simulink model "DYNctl_ver4_etud_nonlineaire_plaque"  (R2014b)
settings: Solver=ode45  StartTime=0.0  StopTime=tfin  FixedStep=0.001  RelTol=1e-09
values from neighbouring files (symbols this model uses):
  ae = sym('ae',[4 1])    [MatlabProjet.m]    (also in bancEssaiConstantes.m = [1.3463 349.0774 1450.3848 703344.2113]; bancessai_ini.m)
  as = sym('as',[4 1])    [MatlabProjet.m]    (also in bancEssaiConstantes.m = [0.052961 30.5716 -1152.4168 344545.4587]; bancessai_ini.m)
  b_E1 = 13.029359254409743    (= 13.0293592544)    [MatlabProjet.m]    (also in bancEssaiConstantes.m; bancessai_ini.m)
  g = 9.81    [MatlabProjet.m]    (also in bancEssaiConstantes.m; bancessai_ini.m; trajectoire.m = sqrt(1 + dy.^2))
  Ixy = 0.0011691    [MatlabProjet.m]    (also in bancEssaiConstantes.m; bancessai_ini.m)
  L_bobine = 115    [MatlabProjet.m]    (also in bancEssaiConstantes.m = 0.115; bancessai_ini.m)
  mS = 0.0080*sig    [bancEssaiConstantes.m]
  mtot = mP + sig*mS    [bancEssaiConstantes.m]
  Pzeq = .015    (= 0.015)    [run_bancessai.m]
  R_bobine = 3.6    [MatlabProjet.m]    (also in bancEssaiConstantes.m; bancessai_ini.m)
  rABC = 95.20e-03    (= 0.0952)    [bancEssaiConstantes.m]
  Va_eq = R_bobine * Ia_eq    [MatlabEquilibre.m]    (also in bancessai_ini.m = Ia_eq*R_bobine; equilibre.m = Ia_eq*R_bobine)
  Vb_eq = R_bobine * Ib_eq    [MatlabEquilibre.m]    (also in bancessai_ini.m = Ib_eq*R_bobine; equilibre.m = Ib_eq*R_bobine)
  Vc_eq = R_bobine * Ic_eq    [MatlabEquilibre.m]    (also in bancessai_ini.m = Ic_eq*R_bobine; equilibre.m = Ic_eq*R_bobine)
  XA = r_ABC    (= 0.0952)    [MatlabProjet.m]    (also in bancEssaiConstantes.m; bancessai_ini.m)
  XB = -r_ABC*sind(30)    [MatlabProjet.m]    (also in bancEssaiConstantes.m = -rABC*sind(30); bancessai_ini.m)
  XC = XB    [MatlabProjet.m]    (also in bancEssaiConstantes.m = -rABC*sind(30); bancessai_ini.m)
  XD = r_DEF*sind(30)    [MatlabProjet.m]    (also in bancEssaiConstantes.m = +rDEF*sind(30); bancessai_ini.m)
  XE = -r_DEF    (= -0.08)    [MatlabProjet.m]    (also in bancEssaiConstantes.m; bancessai_ini.m)
  XF = XD    [MatlabProjet.m]    (also in bancEssaiConstantes.m = +rDEF*sind(30); bancessai_ini.m)
  YA = 0    [MatlabProjet.m]    (also in bancEssaiConstantes.m; bancessai_ini.m)
  YB = r_ABC*cosd(30)    [MatlabProjet.m]    (also in bancEssaiConstantes.m = +rABC*cosd(30); bancessai_ini.m)
  YC = -YB    [MatlabProjet.m]    (also in bancEssaiConstantes.m = -rABC*cosd(30); bancessai_ini.m)
  YD = r_DEF*cosd(30)    [MatlabProjet.m]    (also in bancEssaiConstantes.m = +rDEF*cosd(30); bancessai_ini.m)
  YE = 0    [MatlabProjet.m]    (also in bancEssaiConstantes.m; bancessai_ini.m)
  YF = -YD    [MatlabProjet.m]    (also in bancEssaiConstantes.m = -rDEF*cosd(30); bancessai_ini.m)
undefined symbols (not defined in the file or in its folder): den_pt, den_z, num_pt, num_z, sym2poly
settings Model: Creator=delafontaine  LastModifiedBy=lemg2013
settings SolverCC: AlgebraicLoopSolver=LineSearch
settings DataIOCC: SignalLoggingSaveFormat=ModelDataLogs
settings DebuggingCC: UnderspecifiedInitializationDetection=Classic  MergeDetectMultiDrivingBlocksExec=none  SolverPrmCheckMsg=none  MultiTaskDSMMsg=warning  MultiTaskCondExecSysMsg=none  FrameProcessingCompatibilityMsg=error
settings RTWCC: IncludeERTFirstTime=on

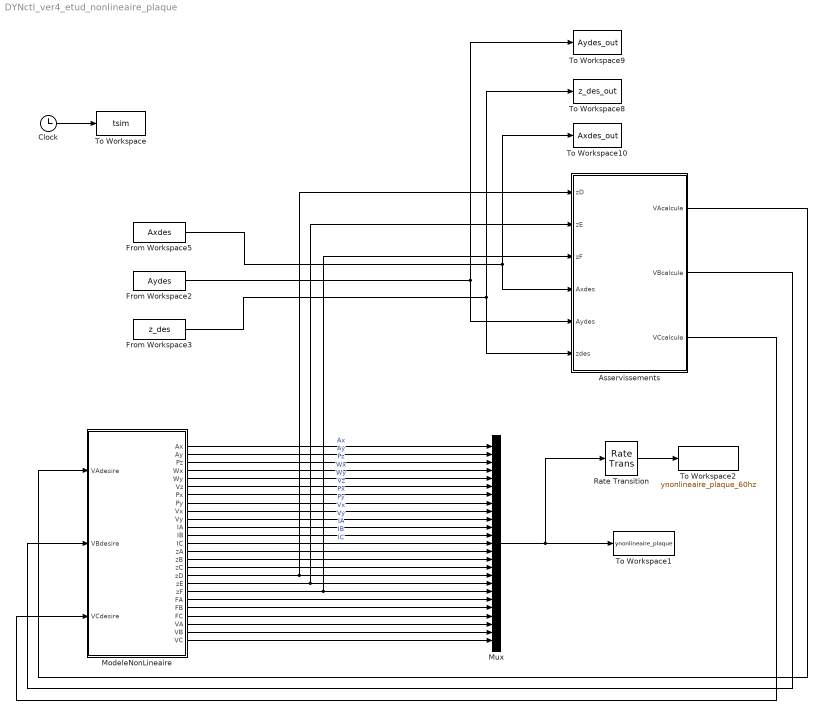
== system DYNctl_ver4_etud_nonlineaire_plaque ==
  Asservissements : Subsystem
      mask help: Simulink:masks:GenSFuncDesc_MD
      mask Help: eval('feval(''rtwprivate'',''rtwhelpview'',''rtw_sfcn_block'')');
  Clock : Clock
  From Workspace2 : FromWorkspace  VariableName=Aydes  SampleTime=0  Interpolate=off  OutputAfterFinalValue=Holding final value
  From Workspace3 : FromWorkspace  VariableName=z_des  SampleTime=0  Interpolate=off  OutputAfterFinalValue=Holding final value
  From Workspace5 : FromWorkspace  VariableName=Axdes  SampleTime=0  Interpolate=off  OutputAfterFinalValue=Holding final value
  ModeleNonLineaire : Subsystem
      mask help: Simulink:masks:GenSFuncDesc_MD
      mask Help: eval('feval(''rtwprivate'',''rtwhelpview'',''rtw_sfcn_block'')');
  Mux : Mux  Inputs=25
  Rate Transition : RateTransition  OutPortSampleTime=1/60
  To Workspace : ToWorkspace  VariableName=tsim  SampleTime=-1
  To Workspace1 : ToWorkspace  VariableName=ynonlineaire_plaque  SampleTime=-1
  To Workspace10 : ToWorkspace  VariableName=Axdes_out  SampleTime=-1
  To Workspace2 : ToWorkspace  VariableName=ynonlineaire_plaque_60hz  SampleTime=-1
  To Workspace8 : ToWorkspace  VariableName=z_des_out  SampleTime=-1
  To Workspace9 : ToWorkspace  VariableName=Aydes_out  SampleTime=-1
  wires:
  Clock/1 -> To Workspace/1
  From Workspace5/1 -> Asservissements/4(Axdes), To Workspace10/1
  ModeleNonLineaire/1(Ax) -> Mux/1  "Ax"
  ModeleNonLineaire/2(Ay) -> Mux/2  "Ay"
  ModeleNonLineaire/3(Pz) -> Mux/3  "Pz"
  ModeleNonLineaire/4(Wx) -> Mux/4  "Wx"
  ModeleNonLineaire/5(Wy) -> Mux/5  "Wy"
  ModeleNonLineaire/6(Vz) -> Mux/6  "Vz"
  ModeleNonLineaire/7(Px) -> Mux/7  "Px"
  ModeleNonLineaire/8(Py) -> Mux/8  "Py"
  ModeleNonLineaire/9(Vx) -> Mux/9  "Vx"
  ModeleNonLineaire/10(Vy) -> Mux/10  "Vy"
  ModeleNonLineaire/11(IA) -> Mux/11  "IA"
  ModeleNonLineaire/12(IB) -> Mux/12  "IB"
  ModeleNonLineaire/13(IC) -> Mux/13  "IC"
  From Workspace3/1 -> Asservissements/6(zdes), To Workspace8/1
  From Workspace2/1 -> Asservissements/5(Aydes), To Workspace9/1
  ModeleNonLineaire/20(FA) -> Mux/20
  ModeleNonLineaire/21(FB) -> Mux/21
  ModeleNonLineaire/22(FC) -> Mux/22
  ModeleNonLineaire/23(VA) -> Mux/23
  ModeleNonLineaire/24(VB) -> Mux/24
  ModeleNonLineaire/25(VC) -> Mux/25
  ModeleNonLineaire/17(zD) -> Asservissements/1(zD), Mux/17
  ModeleNonLineaire/18(zE) -> Asservissements/2(zE), Mux/18
  ModeleNonLineaire/19(zF) -> Asservissements/3(zF), Mux/19
  ModeleNonLineaire/14(zA) -> Mux/14
  ModeleNonLineaire/15(zB) -> Mux/15
  ModeleNonLineaire/16(zC) -> Mux/16
  Asservissements/1(VAcalcule) -> ModeleNonLineaire/1(VAdesire)
  Asservissements/2(VBcalcule) -> ModeleNonLineaire/2(VBdesire)
  Asservissements/3(VCcalcule) -> ModeleNonLineaire/3(VCdesire)
  Mux/1 -> Rate Transition/1, To Workspace1/1
  Rate Transition/1 -> To Workspace2/1

== system DYNctl_ver4_etud_nonlineaire_plaque/Asservissements ==
  zD : Inport
  zE : Inport  Port=2
  zF : Inport  Port=3
  Axdes : Inport  Port=4
  Aydes : Inport  Port=5
  zdes : Inport  Port=6
  Asservissements_fc : Subsystem
  __InputSSForSFun__ : Subsystem
  __OutputSSForSFun__ : Subsystem
  VAcalcule : Outport
  VBcalcule : Outport  Port=2
  VCcalcule : Outport  Port=3
  wires:
  zD/1 -> __InputSSForSFun__/1(zD)
  zE/1 -> __InputSSForSFun__/2(zE)
  zF/1 -> __InputSSForSFun__/3(zF)
  Axdes/1 -> __InputSSForSFun__/4(Axdes)
  Aydes/1 -> __InputSSForSFun__/5(Aydes)
  zdes/1 -> __InputSSForSFun__/6(zdes)
  __InputSSForSFun__/1(__UniqueOutportName__1__) -> Asservissements_fc/1(zD)
  __InputSSForSFun__/2(__UniqueOutportName__2__) -> Asservissements_fc/2(zE)
  __InputSSForSFun__/3(__UniqueOutportName__3__) -> Asservissements_fc/3(zF)
  __InputSSForSFun__/4(__UniqueOutportName__4__) -> Asservissements_fc/4(Axdes)
  __InputSSForSFun__/5(__UniqueOutportName__5__) -> Asservissements_fc/5(Aydes)
  __InputSSForSFun__/6(__UniqueOutportName__6__) -> Asservissements_fc/6(zdes)
  Asservissements_fc/1(Vacalc) -> __OutputSSForSFun__/1(__UniqueInportName__1__)
  Asservissements_fc/2(Vbcalc) -> __OutputSSForSFun__/2(__UniqueInportName__2__)
  Asservissements_fc/3(Vccalc) -> __OutputSSForSFun__/3(__UniqueInportName__3__)
  __OutputSSForSFun__/1(VAcalcule) -> VAcalcule/1
  __OutputSSForSFun__/2(VBcalcule) -> VBcalcule/1
  __OutputSSForSFun__/3(VCcalcule) -> VCcalcule/1

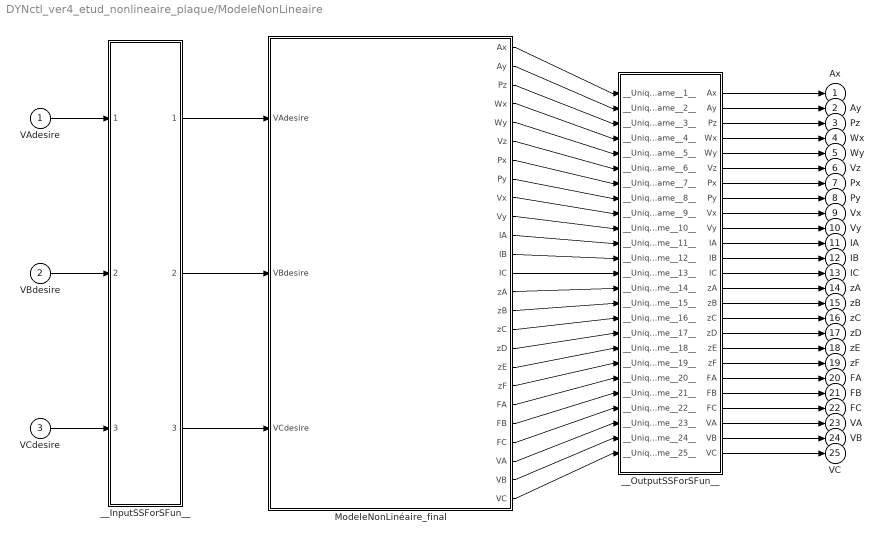
== system DYNctl_ver4_etud_nonlineaire_plaque/ModeleNonLineaire ==
  VAdesire : Inport
  VBdesire : Inport  Port=2
  VCdesire : Inport  Port=3
  ModeleNonLinéaire_final : Subsystem
  __InputSSForSFun__ : Subsystem
  __OutputSSForSFun__ : Subsystem
  Ax : Outport
  Ay : Outport  Port=2
  Pz : Outport  Port=3
  Wx : Outport  Port=4
  Wy : Outport  Port=5
  Vz : Outport  Port=6
  Px : Outport  Port=7
  Py : Outport  Port=8
  Vx : Outport  Port=9
  Vy : Outport  Port=10
  IA : Outport  Port=11
  IB : Outport  Port=12
  IC : Outport  Port=13
  zA : Outport  Port=14
  zB : Outport  Port=15
  zC : Outport  Port=16
  zD : Outport  Port=17
  zE : Outport  Port=18
  zF : Outport  Port=19
  FA : Outport  Port=20
  FB : Outport  Port=21
  FC : Outport  Port=22
  VA : Outport  Port=23
  VB : Outport  Port=24
  VC : Outport  Port=25
  wires:
  VAdesire/1 -> __InputSSForSFun__/1(VAdesire)
  VBdesire/1 -> __InputSSForSFun__/2(VBdesire)
  VCdesire/1 -> __InputSSForSFun__/3(VCdesire)
  __InputSSForSFun__/1(__UniqueOutportName__1__) -> ModeleNonLinéaire_final/1(VAdesire)
  ModeleNonLinéaire_final/1(Ax) -> __OutputSSForSFun__/1(__UniqueInportName__1__)
  ModeleNonLinéaire_final/2(Ay) -> __OutputSSForSFun__/2(__UniqueInportName__2__)
  ModeleNonLinéaire_final/3(Pz) -> __OutputSSForSFun__/3(__UniqueInportName__3__)
  ModeleNonLinéaire_final/4(Wx) -> __OutputSSForSFun__/4(__UniqueInportName__4__)
  ModeleNonLinéaire_final/5(Wy) -> __OutputSSForSFun__/5(__UniqueInportName__5__)
  ModeleNonLinéaire_final/6(Vz) -> __OutputSSForSFun__/6(__UniqueInportName__6__)
  ModeleNonLinéaire_final/7(Px) -> __OutputSSForSFun__/7(__UniqueInportName__7__)
  ModeleNonLinéaire_final/8(Py) -> __OutputSSForSFun__/8(__UniqueInportName__8__)
  ModeleNonLinéaire_final/9(Vx) -> __OutputSSForSFun__/9(__UniqueInportName__9__)
  ModeleNonLinéaire_final/10(Vy) -> __OutputSSForSFun__/10(__UniqueInportName__10__)
  ModeleNonLinéaire_final/11(IA) -> __OutputSSForSFun__/11(__UniqueInportName__11__)
  ModeleNonLinéaire_final/12(IB) -> __OutputSSForSFun__/12(__UniqueInportName__12__)
  ModeleNonLinéaire_final/13(IC) -> __OutputSSForSFun__/13(__UniqueInportName__13__)
  ModeleNonLinéaire_final/14(zA) -> __OutputSSForSFun__/14(__UniqueInportName__14__)
  ModeleNonLinéaire_final/15(zB) -> __OutputSSForSFun__/15(__UniqueInportName__15__)
  ModeleNonLinéaire_final/16(zC) -> __OutputSSForSFun__/16(__UniqueInportName__16__)
  ModeleNonLinéaire_final/17(zD) -> __OutputSSForSFun__/17(__UniqueInportName__17__)
  ModeleNonLinéaire_final/18(zE) -> __OutputSSForSFun__/18(__UniqueInportName__18__)
  ModeleNonLinéaire_final/19(zF) -> __OutputSSForSFun__/19(__UniqueInportName__19__)
  ModeleNonLinéaire_final/20(FA) -> __OutputSSForSFun__/20(__UniqueInportName__20__)
  ModeleNonLinéaire_final/21(FB) -> __OutputSSForSFun__/21(__UniqueInportName__21__)
  ModeleNonLinéaire_final/22(FC) -> __OutputSSForSFun__/22(__UniqueInportName__22__)
  ModeleNonLinéaire_final/23(VA) -> __OutputSSForSFun__/23(__UniqueInportName__23__)
  ModeleNonLinéaire_final/24(VB) -> __OutputSSForSFun__/24(__UniqueInportName__24__)
  ModeleNonLinéaire_final/25(VC) -> __OutputSSForSFun__/25(__UniqueInportName__25__)
  __OutputSSForSFun__/1(Ax) -> Ax/1
  __OutputSSForSFun__/2(Ay) -> Ay/1
  __OutputSSForSFun__/3(Pz) -> Pz/1
  __OutputSSForSFun__/4(Wx) -> Wx/1
  __OutputSSForSFun__/5(Wy) -> Wy/1
  __OutputSSForSFun__/6(Vz) -> Vz/1
  __OutputSSForSFun__/7(Px) -> Px/1
  __OutputSSForSFun__/8(Py) -> Py/1
  __OutputSSForSFun__/9(Vx) -> Vx/1
  __OutputSSForSFun__/10(Vy) -> Vy/1
  __OutputSSForSFun__/11(IA) -> IA/1
  __OutputSSForSFun__/12(IB) -> IB/1
  __OutputSSForSFun__/13(IC) -> IC/1
  __OutputSSForSFun__/14(zA) -> zA/1
  __OutputSSForSFun__/15(zB) -> zB/1
  __OutputSSForSFun__/16(zC) -> zC/1
  __OutputSSForSFun__/17(zD) -> zD/1
  __OutputSSForSFun__/18(zE) -> zE/1
  __OutputSSForSFun__/19(zF) -> zF/1
  __OutputSSForSFun__/20(FA) -> FA/1
  __OutputSSForSFun__/21(FB) -> FB/1
  __OutputSSForSFun__/22(FC) -> FC/1
  __OutputSSForSFun__/23(VA) -> VA/1
  __OutputSSForSFun__/24(VB) -> VB/1
  __OutputSSForSFun__/25(VC) -> VC/1
  __InputSSForSFun__/2(__UniqueOutportName__2__) -> ModeleNonLinéaire_final/2(VBdesire)
  __InputSSForSFun__/3(__UniqueOutportName__3__) -> ModeleNonLinéaire_final/3(VCdesire)

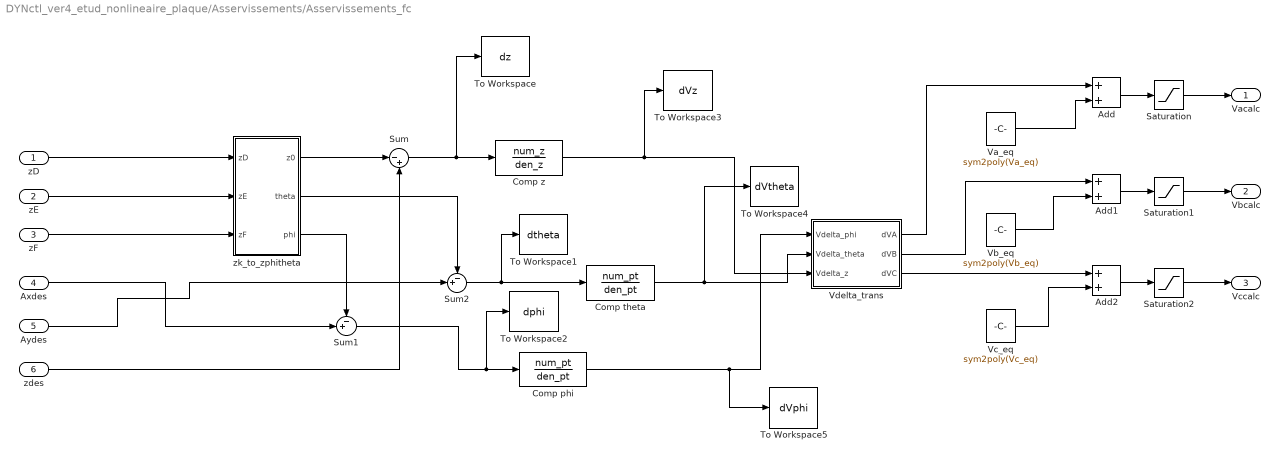
== system DYNctl_ver4_etud_nonlineaire_plaque/Asservissements/Asservissements_fc ==
  zD : Inport
  zE : Inport  Port=2
  zF : Inport  Port=3
  Axdes : Inport  Port=4
  Aydes : Inport  Port=5
  zdes : Inport  Port=6
  Add : Sum
  Add1 : Sum
  Add2 : Sum
  Comp phi : TransferFcn  Numerator=num_pt  Denominator=den_pt
  Comp theta : TransferFcn  Numerator=num_pt  Denominator=den_pt
  Comp z : TransferFcn  Numerator=num_z  Denominator=den_z
  Saturation : Saturate  UpperLimit=22  LowerLimit=-22
  Saturation1 : Saturate  UpperLimit=22  LowerLimit=-22
  Saturation2 : Saturate  UpperLimit=22  LowerLimit=-22
  Sum : Sum  Inputs=|-+
  Sum1 : Sum  Inputs=-+|
  Sum2 : Sum  Inputs=-+|
  To Workspace : ToWorkspace  VariableName=dz  SampleTime=-1
      settings: Save2DSignal=2-D array (concatenate along first dimension)
  To Workspace1 : ToWorkspace  VariableName=dtheta  SampleTime=-1
      settings: Save2DSignal=2-D array (concatenate along first dimension)
  To Workspace2 : ToWorkspace  VariableName=dphi  SampleTime=-1
      settings: Save2DSignal=2-D array (concatenate along first dimension)
  To Workspace3 : ToWorkspace  VariableName=dVz  SampleTime=-1
      settings: Save2DSignal=2-D array (concatenate along first dimension)
  To Workspace4 : ToWorkspace  VariableName=dVtheta  SampleTime=-1
      settings: Save2DSignal=2-D array (concatenate along first dimension)
  To Workspace5 : ToWorkspace  VariableName=dVphi  SampleTime=-1
      settings: Save2DSignal=2-D array (concatenate along first dimension)
  Va_eq : Constant  Value=sym2poly(Va_eq)  VectorParams1D=off
  Vb_eq : Constant  Value=sym2poly(Vb_eq)  VectorParams1D=off
  Vc_eq : Constant  Value=sym2poly(Vc_eq)  VectorParams1D=off
  Vdelta_trans : Subsystem
  zk_to_zphitheta : Subsystem
  Vacalc : Outport
  Vbcalc : Outport  Port=2
  Vccalc : Outport  Port=3
  wires:
  zD/1 -> zk_to_zphitheta/1(zD)
  zE/1 -> zk_to_zphitheta/2(zE)
  zF/1 -> zk_to_zphitheta/3(zF)
  zdes/1 -> Sum/2
  zk_to_zphitheta/1(z0) -> Sum/1
  Sum/1 -> To Workspace/1, Comp z/1
  Comp z/1 -> To Workspace3/1, Vdelta_trans/3(Vdelta_z)
  zk_to_zphitheta/3(phi) -> Sum1/1
  zk_to_zphitheta/2(theta) -> Sum2/1
  Vdelta_trans/3(dVC) -> Add2/1
  Sum1/1 -> Comp phi/1, To Workspace2/1
  Sum2/1 -> To Workspace1/1, Comp theta/1
  Comp phi/1 -> To Workspace5/1, Vdelta_trans/1(Vdelta_phi)
  Vdelta_trans/1(dVA) -> Add/1
  Vdelta_trans/2(dVB) -> Add1/1
  Comp theta/1 -> To Workspace4/1, Vdelta_trans/2(Vdelta_theta)
  Add/1 -> Saturation/1
  Add1/1 -> Saturation1/1
  Add2/1 -> Saturation2/1
  Va_eq/1 -> Add/2
  Vc_eq/1 -> Add2/2
  Vb_eq/1 -> Add1/2
  Axdes/1 -> Sum1/2
  Aydes/1 -> Sum2/2
  Saturation/1 -> Vacalc/1
  Saturation1/1 -> Vbcalc/1
  Saturation2/1 -> Vccalc/1

== system DYNctl_ver4_etud_nonlineaire_plaque/Asservissements/__InputSSForSFun__ ==
  zD : Inport
  zE : Inport  Port=2
  zF : Inport  Port=3
  Axdes : Inport  Port=4
  Aydes : Inport  Port=5
  zdes : Inport  Port=6
  __UniqueOutportName__1__ : Outport
  __UniqueOutportName__2__ : Outport  Port=2
  __UniqueOutportName__3__ : Outport  Port=3
  __UniqueOutportName__4__ : Outport  Port=4
  __UniqueOutportName__5__ : Outport  Port=5
  __UniqueOutportName__6__ : Outport  Port=6
  wires:
  zD/1 -> __UniqueOutportName__1__/1
  zE/1 -> __UniqueOutportName__2__/1
  zF/1 -> __UniqueOutportName__3__/1
  Axdes/1 -> __UniqueOutportName__4__/1
  Aydes/1 -> __UniqueOutportName__5__/1
  zdes/1 -> __UniqueOutportName__6__/1

== system DYNctl_ver4_etud_nonlineaire_plaque/Asservissements/__OutputSSForSFun__ ==
  __UniqueInportName__1__ : Inport
  __UniqueInportName__2__ : Inport  Port=2
  __UniqueInportName__3__ : Inport  Port=3
  VAcalcule : Outport
  VBcalcule : Outport  Port=2
  VCcalcule : Outport  Port=3
  wires:
  __UniqueInportName__1__/1 -> VAcalcule/1
  __UniqueInportName__2__/1 -> VBcalcule/1
  __UniqueInportName__3__/1 -> VCcalcule/1

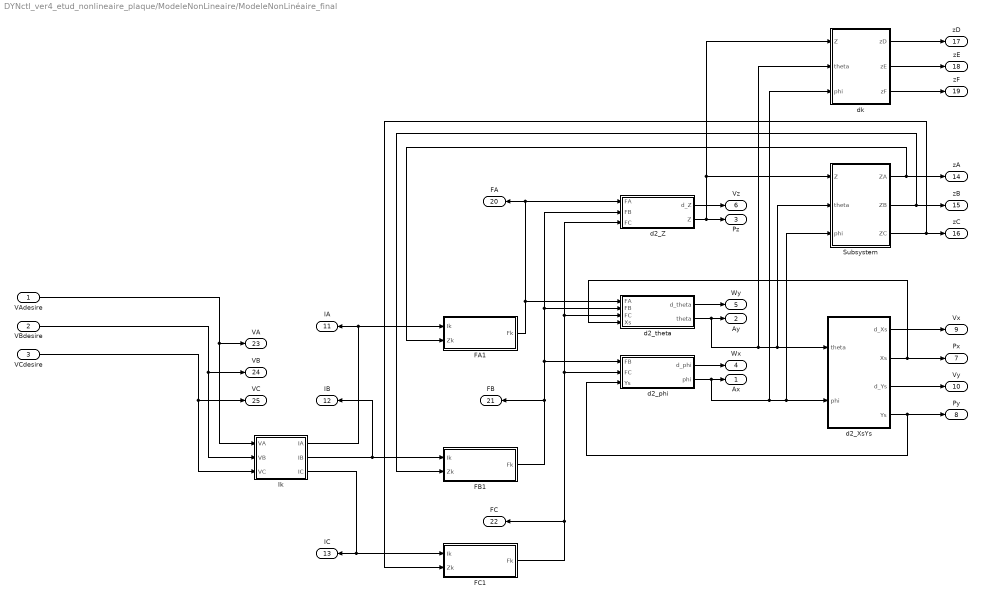
== system DYNctl_ver4_etud_nonlineaire_plaque/ModeleNonLineaire/ModeleNonLinéaire_final ==
  VAdesire : Inport
  VBdesire : Inport  Port=2
  VCdesire : Inport  Port=3
  FA1 : Subsystem
  FB1 : Subsystem
  FC1 : Subsystem
  Ik : Subsystem
  Subsystem : Subsystem
  d2_XsYs : Subsystem
  d2_Z : Subsystem
  d2_phi : Subsystem
  d2_theta : Subsystem
  dk : Subsystem
  Ax : Outport
  Ay : Outport  Port=2
  Pz : Outport  Port=3
  Wx : Outport  Port=4
  Wy : Outport  Port=5
  Vz : Outport  Port=6
  Px : Outport  Port=7
  Py : Outport  Port=8
  Vx : Outport  Port=9
  Vy : Outport  Port=10
  IA : Outport  Port=11
  IB : Outport  Port=12
  IC : Outport  Port=13
  zA : Outport  Port=14
  zB : Outport  Port=15
  zC : Outport  Port=16
  zD : Outport  Port=17
  zE : Outport  Port=18
  zF : Outport  Port=19
  FA : Outport  Port=20
  FB : Outport  Port=21
  FC : Outport  Port=22
  VA : Outport  Port=23
  VB : Outport  Port=24
  VC : Outport  Port=25
  wires:
  VAdesire/1 -> Ik/1(VA), VA/1
  VBdesire/1 -> VB/1, Ik/2(VB)
  VCdesire/1 -> Ik/3(VC), VC/1
  Ik/1(IA) -> IA/1, FA1/1(Ik)
  Ik/2(IB) -> IB/1, FB1/1(Ik)
  Ik/3(IC) -> FC1/1(Ik), IC/1
  FA1/1(Fk) -> FA/1, d2_Z/1(FA), d2_theta/1(FA)
  FB1/1(Fk) -> d2_phi/1(FB), d2_Z/2(FB), d2_theta/2(FB), FB/1
  FC1/1(Fk) -> d2_Z/3(FC), d2_theta/3(FC), d2_phi/2(FC), FC/1
  d2_phi/2("phi ") -> Ax/1, dk/3(phi), Subsystem/3(phi), d2_XsYs/2(phi)
  d2_theta/2("theta ") -> Ay/1, dk/2(theta), Subsystem/2(theta), d2_XsYs/1(theta)
  d2_XsYs/2(Xs) -> d2_theta/4(Xs), Px/1
  d2_XsYs/4(Ys) -> Py/1, d2_phi/3(Ys)
  d2_Z/2(Z) -> dk/1(Z), Subsystem/1(Z), Pz/1
  Subsystem/1(ZA) -> FA1/2(Zk), zA/1
  Subsystem/2(ZB) -> FB1/2(Zk), zB/1
  Subsystem/3(ZC) -> FC1/2(Zk), zC/1
  d2_phi/1("d_phi ") -> Wx/1
  d2_theta/1("d_theta ") -> Wy/1
  d2_Z/1(d_Z) -> Vz/1
  d2_XsYs/1(d_Xs) -> Vx/1
  d2_XsYs/3(d_Ys) -> Vy/1
  dk/1(zD) -> zD/1
  dk/2(zE) -> zE/1
  dk/3(zF) -> zF/1

== system DYNctl_ver4_etud_nonlineaire_plaque/ModeleNonLineaire/__InputSSForSFun__ ==
  VAdesire : Inport
  VBdesire : Inport  Port=2
  VCdesire : Inport  Port=3
  __UniqueOutportName__1__ : Outport
  __UniqueOutportName__2__ : Outport  Port=2
  __UniqueOutportName__3__ : Outport  Port=3
  wires:
  VAdesire/1 -> __UniqueOutportName__1__/1
  VBdesire/1 -> __UniqueOutportName__2__/1
  VCdesire/1 -> __UniqueOutportName__3__/1

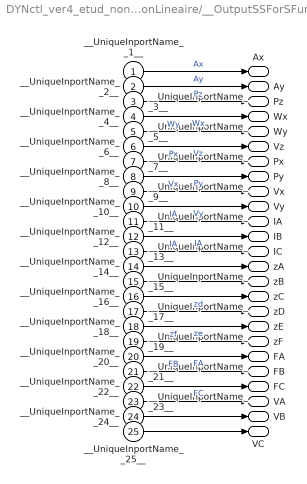
== system DYNctl_ver4_etud_nonlineaire_plaque/ModeleNonLineaire/__OutputSSForSFun__ ==
  __UniqueInportName__1__ : Inport
  __UniqueInportName__2__ : Inport  Port=2
  __UniqueInportName__3__ : Inport  Port=3
  __UniqueInportName__4__ : Inport  Port=4
  __UniqueInportName__5__ : Inport  Port=5
  __UniqueInportName__6__ : Inport  Port=6
  __UniqueInportName__7__ : Inport  Port=7
  __UniqueInportName__8__ : Inport  Port=8
  __UniqueInportName__9__ : Inport  Port=9
  __UniqueInportName__10__ : Inport  Port=10
  __UniqueInportName__11__ : Inport  Port=11
  __UniqueInportName__12__ : Inport  Port=12
  __UniqueInportName__13__ : Inport  Port=13
  __UniqueInportName__14__ : Inport  Port=14
  __UniqueInportName__15__ : Inport  Port=15
  __UniqueInportName__16__ : Inport  Port=16
  __UniqueInportName__17__ : Inport  Port=17
  __UniqueInportName__18__ : Inport  Port=18
  __UniqueInportName__19__ : Inport  Port=19
  __UniqueInportName__20__ : Inport  Port=20
  __UniqueInportName__21__ : Inport  Port=21
  __UniqueInportName__22__ : Inport  Port=22
  __UniqueInportName__23__ : Inport  Port=23
  __UniqueInportName__24__ : Inport  Port=24
  __UniqueInportName__25__ : Inport  Port=25
  Ax : Outport
  Ay : Outport  Port=2
  Pz : Outport  Port=3
  Wx : Outport  Port=4
  Wy : Outport  Port=5
  Vz : Outport  Port=6
  Px : Outport  Port=7
  Py : Outport  Port=8
  Vx : Outport  Port=9
  Vy : Outport  Port=10
  IA : Outport  Port=11
  IB : Outport  Port=12
  IC : Outport  Port=13
  zA : Outport  Port=14
  zB : Outport  Port=15
  zC : Outport  Port=16
  zD : Outport  Port=17
  zE : Outport  Port=18
  zF : Outport  Port=19
  FA : Outport  Port=20
  FB : Outport  Port=21
  FC : Outport  Port=22
  VA : Outport  Port=23
  VB : Outport  Port=24
  VC : Outport  Port=25
  wires:
  __UniqueInportName__1__/1 -> Ax/1  "Ax"
  __UniqueInportName__2__/1 -> Ay/1  "Ay"
  __UniqueInportName__3__/1 -> Pz/1  "Pz"
  __UniqueInportName__4__/1 -> Wx/1  "Wx"
  __UniqueInportName__5__/1 -> Wy/1  "Wy"
  __UniqueInportName__6__/1 -> Vz/1  "Vz"
  __UniqueInportName__7__/1 -> Px/1  "Px"
  __UniqueInportName__8__/1 -> Py/1  "Py"
  __UniqueInportName__9__/1 -> Vx/1  "Vx"
  __UniqueInportName__10__/1 -> Vy/1  "Vy"
  __UniqueInportName__11__/1 -> IA/1  "IA"
  __UniqueInportName__12__/1 -> IB/1  "IA"
  __UniqueInportName__13__/1 -> IC/1  "IA"
  __UniqueInportName__14__/1 -> zA/1
  __UniqueInportName__15__/1 -> zB/1
  __UniqueInportName__16__/1 -> zC/1
  __UniqueInportName__17__/1 -> zD/1  "zd"
  __UniqueInportName__18__/1 -> zE/1  "ze"
  __UniqueInportName__19__/1 -> zF/1  "zf"
  __UniqueInportName__20__/1 -> FA/1  "FA"
  __UniqueInportName__21__/1 -> FB/1  "FB"
  __UniqueInportName__22__/1 -> FC/1  "FC"
  __UniqueInportName__23__/1 -> VA/1
  __UniqueInportName__24__/1 -> VB/1
  __UniqueInportName__25__/1 -> VC/1

== system DYNctl_ver4_etud_nonlineaire_plaque/Asservissements/Asservissements_fc/Vdelta_trans ==
  Vdelta_phi : Inport
  Vdelta_theta : Inport  Port=2
  Vdelta_z : Inport  Port=3
  Demux : Demux  Outputs=3
  Mux : Mux  Inputs=3
  Product : Product  Multiplication=Matrix(*)
  u : Constant  Value=inv(u)  VectorParams1D=off
  dVA : Outport
  dVB : Outport  Port=2
  dVC : Outport  Port=3
  wires:
  u/1 -> Product/1
  Mux/1 -> Product/2
  Demux/1 -> dVA/1
  Demux/2 -> dVB/1
  Demux/3 -> dVC/1
  Product/1 -> Demux/1
  Vdelta_phi/1 -> Mux/1
  Vdelta_theta/1 -> Mux/2
  Vdelta_z/1 -> Mux/3

== system DYNctl_ver4_etud_nonlineaire_plaque/Asservissements/Asservissements_fc/zk_to_zphitheta ==
  zD : Inport
  zE : Inport  Port=2
  zF : Inport  Port=3
  Add : Sum  Inputs=+++
  Constant : Constant  Value=3
  Constant1 : Constant  Value=-XE
  Constant2 : Constant  Value=XD
  Constant3 : Constant  Value=YD
  Divide : Product  Inputs=*/
  Divide1 : Product  Inputs=*/
  Divide2 : Product  Inputs=*/
  Product : Product
  Sum : Sum  Inputs=|+-
  Sum1 : Sum  Inputs=|-++
  z0 : Outport
  theta : Outport  Port=2
  phi : Outport  Port=3
  wires:
  zD/1 -> Sum1/2, Add/1
  zE/1 -> Sum/1, Add/2
  zF/1 -> Add/3
  Add/1 -> Divide/1
  Constant/1 -> Divide/2
  Divide/1 -> Sum1/1, Sum/2, z0/1
  Sum/1 -> Divide1/1
  Constant1/1 -> Divide1/2
  Divide1/1 -> Product/1, theta/1
  Constant2/1 -> Product/2
  Product/1 -> Sum1/3
  Sum1/1 -> Divide2/1
  Constant3/1 -> Divide2/2
  Divide2/1 -> phi/1

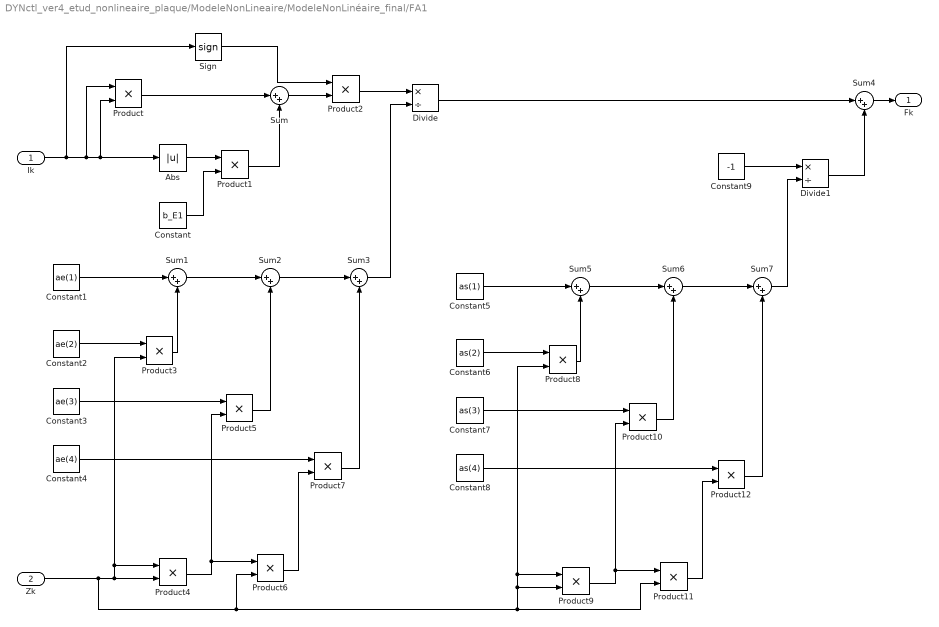
== system DYNctl_ver4_etud_nonlineaire_plaque/ModeleNonLineaire/ModeleNonLinéaire_final/FA1 ==
  Ik : Inport
  Zk : Inport  Port=2
  Abs : Abs
  Constant : Constant  Value=b_E1
  Constant1 : Constant  Value=ae(1)
  Constant2 : Constant  Value=ae(2)
  Constant3 : Constant  Value=ae(3)
  Constant4 : Constant  Value=ae(4)
  Constant5 : Constant  Value=as(1)
  Constant6 : Constant  Value=as(2)
  Constant7 : Constant  Value=as(3)
  Constant8 : Constant  Value=as(4)
  Constant9 : Constant  Value=-1
  Divide : Product  Inputs=*/
  Divide1 : Product  Inputs=*/
  Product{,1..12} (13 alike) : Product
  Sign : Signum
  Sum{,1..7} (8 alike) : Sum  Inputs=|++
  Fk : Outport
  wires:
  Ik/1 -> Sign/1, Product/1, Abs/1, Product/2
  Abs/1 -> Product1/1
  Constant/1 -> Product1/2
  Product1/1 -> Sum/2
  Product/1 -> Sum/1
  Sum/1 -> Product2/2
  Sign/1 -> Product2/1
  Constant1/1 -> Sum1/1
  Constant2/1 -> Product3/1
  Product3/1 -> Sum1/2
  Sum1/1 -> Sum2/1
  Product4/1 -> Product6/1, Product5/2
  Constant3/1 -> Product5/1
  Product5/1 -> Sum2/2
  Constant4/1 -> Product7/1
  Product6/1 -> Product7/2
  Product7/1 -> Sum3/2
  Sum2/1 -> Sum3/1
  Product2/1 -> Divide/1
  Sum3/1 -> Divide/2
  Constant5/1 -> Sum5/1
  Constant6/1 -> Product8/1
  Zk/1 -> Product11/2, Product8/2, Product9/1, Product9/2, Product6/2, Product3/2, Product4/1, Product4/2
  Product8/1 -> Sum5/2
  Sum5/1 -> Sum6/1
  Product9/1 -> Product11/1, Product10/2
  Constant7/1 -> Product10/1
  Product10/1 -> Sum6/2
  Constant8/1 -> Product12/1
  Product11/1 -> Product12/2
  Product12/1 -> Sum7/2
  Sum6/1 -> Sum7/1
  Sum7/1 -> Divide1/2
  Divide/1 -> Sum4/1
  Constant9/1 -> Divide1/1
  Divide1/1 -> Sum4/2
  Sum4/1 -> Fk/1

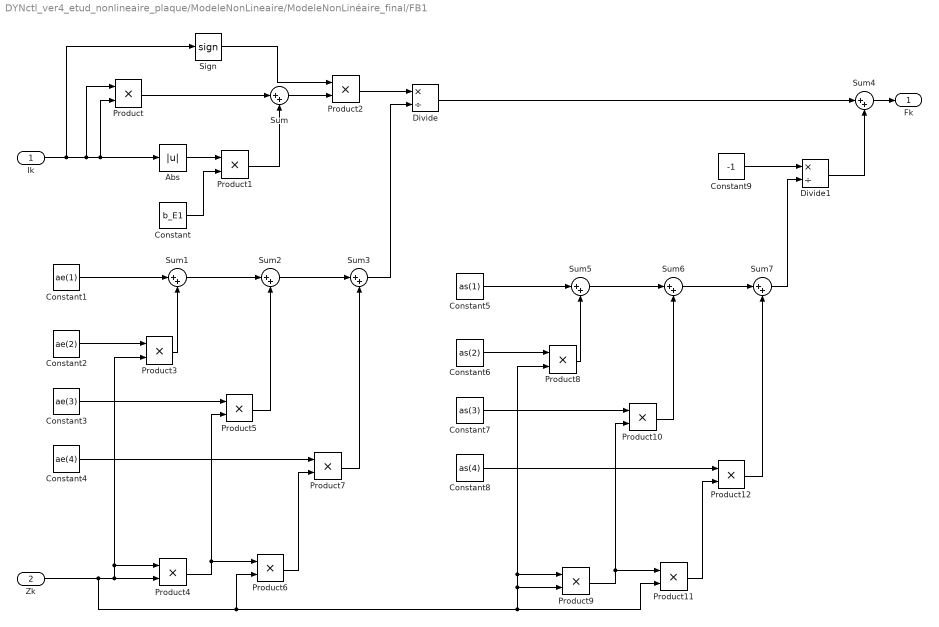
== system DYNctl_ver4_etud_nonlineaire_plaque/ModeleNonLineaire/ModeleNonLinéaire_final/FB1 ==
  Ik : Inport
  Zk : Inport  Port=2
  Abs : Abs
  Constant : Constant  Value=b_E1
  Constant1 : Constant  Value=ae(1)
  Constant2 : Constant  Value=ae(2)
  Constant3 : Constant  Value=ae(3)
  Constant4 : Constant  Value=ae(4)
  Constant5 : Constant  Value=as(1)
  Constant6 : Constant  Value=as(2)
  Constant7 : Constant  Value=as(3)
  Constant8 : Constant  Value=as(4)
  Constant9 : Constant  Value=-1
  Divide : Product  Inputs=*/
  Divide1 : Product  Inputs=*/
  Product{,1..12} (13 alike) : Product
  Sign : Signum
  Sum{,1..7} (8 alike) : Sum  Inputs=|++
  Fk : Outport
  wires:
  Ik/1 -> Sign/1, Product/1, Abs/1, Product/2
  Abs/1 -> Product1/1
  Constant/1 -> Product1/2
  Product1/1 -> Sum/2
  Product/1 -> Sum/1
  Sum/1 -> Product2/2
  Sign/1 -> Product2/1
  Constant1/1 -> Sum1/1
  Constant2/1 -> Product3/1
  Product3/1 -> Sum1/2
  Sum1/1 -> Sum2/1
  Product4/1 -> Product6/1, Product5/2
  Constant3/1 -> Product5/1
  Product5/1 -> Sum2/2
  Constant4/1 -> Product7/1
  Product6/1 -> Product7/2
  Product7/1 -> Sum3/2
  Sum2/1 -> Sum3/1
  Product2/1 -> Divide/1
  Sum3/1 -> Divide/2
  Constant5/1 -> Sum5/1
  Constant6/1 -> Product8/1
  Zk/1 -> Product11/2, Product8/2, Product9/1, Product9/2, Product6/2, Product3/2, Product4/1, Product4/2
  Product8/1 -> Sum5/2
  Sum5/1 -> Sum6/1
  Product9/1 -> Product11/1, Product10/2
  Constant7/1 -> Product10/1
  Product10/1 -> Sum6/2
  Constant8/1 -> Product12/1
  Product11/1 -> Product12/2
  Product12/1 -> Sum7/2
  Sum6/1 -> Sum7/1
  Sum7/1 -> Divide1/2
  Divide/1 -> Sum4/1
  Constant9/1 -> Divide1/1
  Divide1/1 -> Sum4/2
  Sum4/1 -> Fk/1

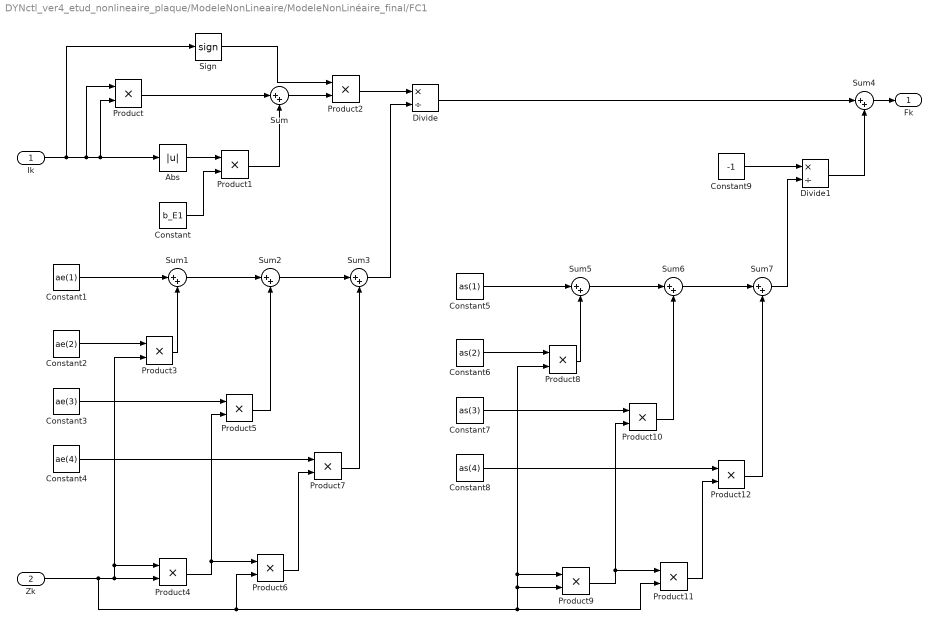
== system DYNctl_ver4_etud_nonlineaire_plaque/ModeleNonLineaire/ModeleNonLinéaire_final/FC1 ==
  Ik : Inport
  Zk : Inport  Port=2
  Abs : Abs
  Constant : Constant  Value=b_E1
  Constant1 : Constant  Value=ae(1)
  Constant2 : Constant  Value=ae(2)
  Constant3 : Constant  Value=ae(3)
  Constant4 : Constant  Value=ae(4)
  Constant5 : Constant  Value=as(1)
  Constant6 : Constant  Value=as(2)
  Constant7 : Constant  Value=as(3)
  Constant8 : Constant  Value=as(4)
  Constant9 : Constant  Value=-1
  Divide : Product  Inputs=*/
  Divide1 : Product  Inputs=*/
  Product{,1..12} (13 alike) : Product
  Sign : Signum
  Sum{,1..7} (8 alike) : Sum  Inputs=|++
  Fk : Outport
  wires:
  Ik/1 -> Sign/1, Product/1, Abs/1, Product/2
  Abs/1 -> Product1/1
  Constant/1 -> Product1/2
  Product1/1 -> Sum/2
  Product/1 -> Sum/1
  Sum/1 -> Product2/2
  Sign/1 -> Product2/1
  Constant1/1 -> Sum1/1
  Constant2/1 -> Product3/1
  Product3/1 -> Sum1/2
  Sum1/1 -> Sum2/1
  Product4/1 -> Product6/1, Product5/2
  Constant3/1 -> Product5/1
  Product5/1 -> Sum2/2
  Constant4/1 -> Product7/1
  Product6/1 -> Product7/2
  Product7/1 -> Sum3/2
  Sum2/1 -> Sum3/1
  Product2/1 -> Divide/1
  Sum3/1 -> Divide/2
  Constant5/1 -> Sum5/1
  Constant6/1 -> Product8/1
  Zk/1 -> Product11/2, Product8/2, Product9/1, Product9/2, Product6/2, Product3/2, Product4/1, Product4/2
  Product8/1 -> Sum5/2
  Sum5/1 -> Sum6/1
  Product9/1 -> Product11/1, Product10/2
  Constant7/1 -> Product10/1
  Product10/1 -> Sum6/2
  Constant8/1 -> Product12/1
  Product11/1 -> Product12/2
  Product12/1 -> Sum7/2
  Sum6/1 -> Sum7/1
  Sum7/1 -> Divide1/2
  Divide/1 -> Sum4/1
  Constant9/1 -> Divide1/1
  Divide1/1 -> Sum4/2
  Sum4/1 -> Fk/1

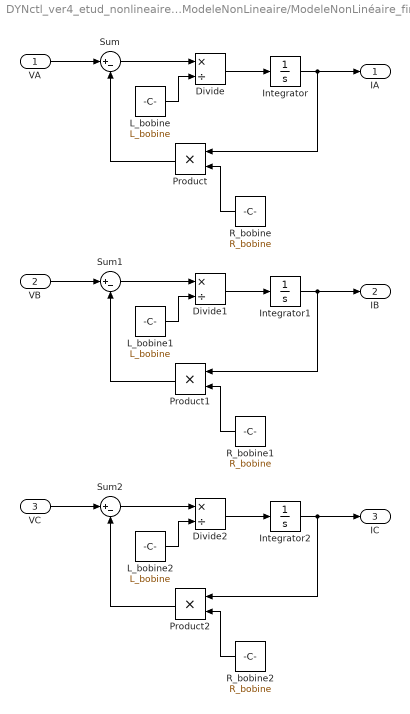
== system DYNctl_ver4_etud_nonlineaire_plaque/ModeleNonLineaire/ModeleNonLinéaire_final/Ik ==
  VA : Inport
  VB : Inport  Port=2
  VC : Inport  Port=3
  Divide : Product  Inputs=*/
  Divide1 : Product  Inputs=*/
  Divide2 : Product  Inputs=*/
  Integrator : Integrator
  Integrator1 : Integrator
  Integrator2 : Integrator
  L_bobine : Constant  Value=L_bobine
  L_bobine1 : Constant  Value=L_bobine
  L_bobine2 : Constant  Value=L_bobine
  Product : Product
  Product1 : Product
  Product2 : Product
  R_bobine : Constant  Value=R_bobine
  R_bobine1 : Constant  Value=R_bobine
  R_bobine2 : Constant  Value=R_bobine
  Sum : Sum  Inputs=|+-
  Sum1 : Sum  Inputs=|+-
  Sum2 : Sum  Inputs=|+-
  IA : Outport
  IB : Outport  Port=2
  IC : Outport  Port=3
  wires:
  Sum/1 -> Divide/1
  L_bobine/1 -> Divide/2
  Divide/1 -> Integrator/1
  Integrator/1 -> IA/1, Product/1
  R_bobine/1 -> Product/2
  Product/1 -> Sum/2
  VA/1 -> Sum/1
  Sum1/1 -> Divide1/1
  L_bobine1/1 -> Divide1/2
  Divide1/1 -> Integrator1/1
  Integrator1/1 -> IB/1, Product1/1
  R_bobine1/1 -> Product1/2
  Product1/1 -> Sum1/2
  VB/1 -> Sum1/1
  Sum2/1 -> Divide2/1
  L_bobine2/1 -> Divide2/2
  Divide2/1 -> Integrator2/1
  Integrator2/1 -> IC/1, Product2/1
  R_bobine2/1 -> Product2/2
  Product2/1 -> Sum2/2
  VC/1 -> Sum2/1

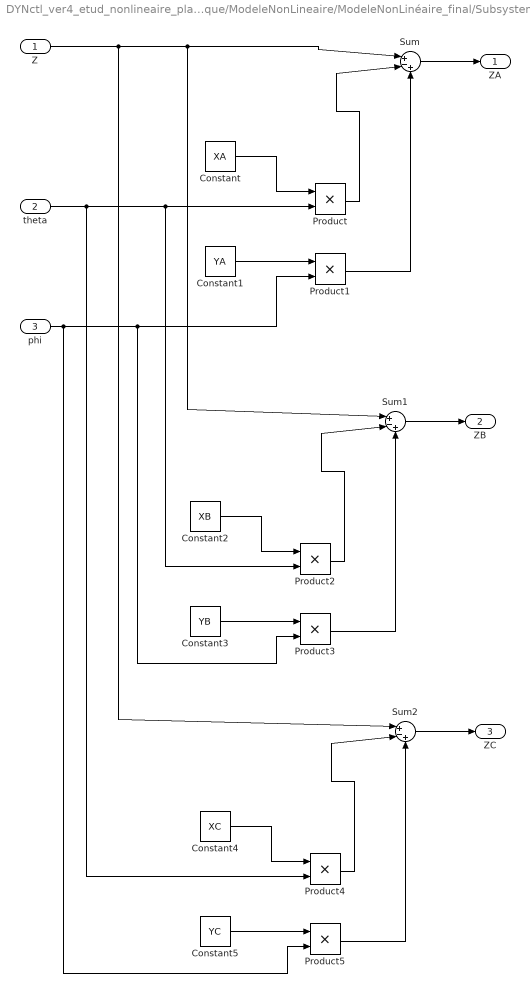
== system DYNctl_ver4_etud_nonlineaire_plaque/ModeleNonLineaire/ModeleNonLinéaire_final/Subsystem ==
  Z : Inport
  theta : Inport  Port=2
  phi : Inport  Port=3
  Constant : Constant  Value=XA
  Constant1 : Constant  Value=YA
  Constant2 : Constant  Value=XB
  Constant3 : Constant  Value=YB
  Constant4 : Constant  Value=XC
  Constant5 : Constant  Value=YC
  Product{,1..5} (6 alike) : Product
  Sum : Sum  Inputs=|+-+
  Sum1 : Sum  Inputs=|+-+
  Sum2 : Sum  Inputs=|+-+
  ZA : Outport
  ZB : Outport  Port=2
  ZC : Outport  Port=3
  wires:
  Constant/1 -> Product/1
  Product/1 -> Sum/2
  Constant1/1 -> Product1/1
  Product1/1 -> Sum/3
  Sum/1 -> ZA/1
  Z/1 -> Sum2/1, Sum1/1, Sum/1
  theta/1 -> Product2/2, Product/2, Product4/2
  Constant2/1 -> Product2/1
  Product2/1 -> Sum1/2
  Constant3/1 -> Product3/1
  phi/1 -> Product3/2, Product1/2, Product5/2
  Product3/1 -> Sum1/3
  Sum1/1 -> ZB/1
  Constant4/1 -> Product4/1
  Product4/1 -> Sum2/2
  Constant5/1 -> Product5/1
  Product5/1 -> Sum2/3
  Sum2/1 -> ZC/1

== system DYNctl_ver4_etud_nonlineaire_plaque/ModeleNonLineaire/ModeleNonLinéaire_final/d2_XsYs ==
  theta : Inport
  phi : Inport  Port=2
  Constant : Constant  Value=-g/1.4
  Constant1 : Constant  Value=g/1.4
  Integrator{,1..3} (4 alike) : Integrator
  Product : Product
  Product1 : Product
  d_Xs : Outport
  Xs : Outport  Port=2
  d_Ys : Outport  Port=3
  Ys : Outport  Port=4
  wires:
  theta/1 -> Product/1
  Constant/1 -> Product/2
  Product/1 -> Integrator/1
  Integrator/1 -> d_Xs/1, Integrator1/1
  Integrator1/1 -> Xs/1
  phi/1 -> Product1/1
  Constant1/1 -> Product1/2
  Product1/1 -> Integrator2/1
  Integrator2/1 -> d_Ys/1, Integrator3/1
  Integrator3/1 -> Ys/1

== system DYNctl_ver4_etud_nonlineaire_plaque/ModeleNonLineaire/ModeleNonLinéaire_final/d2_Z ==
  FA : Inport
  FB : Inport  Port=2
  FC : Inport  Port=3
  Constant : Constant  Value=mtot
  Constant1 : Constant  Value=g
  Divide : Product  Inputs=*/
  Integrator : Integrator
  Integrator1 : Integrator  InitialCondition=Pzeq
  Product : Product
  Sum : Sum  Inputs=++++
  d_Z : Outport
  Z : Outport  Port=2
  wires:
  FB/1 -> Sum/2
  FA/1 -> Sum/1
  FC/1 -> Sum/3
  Constant1/1 -> Product/2
  Product/1 -> Sum/4
  Sum/1 -> Divide/1
  Constant/1 -> Divide/2, Product/1
  Divide/1 -> Integrator/1
  Integrator1/1 -> Z/1
  Integrator/1 -> Integrator1/1, d_Z/1

== system DYNctl_ver4_etud_nonlineaire_plaque/ModeleNonLineaire/ModeleNonLinéaire_final/d2_phi ==
  FB : Inport
  FC : Inport  Port=2
  Ys : Inport  Port=3
  Constant : Constant  Value=Ixy
  Divide : Product  Inputs=*/
  Integrator : Integrator
  Integrator1 : Integrator
  Product{,1..4} (5 alike) : Product
  Sum : Sum  Inputs=|+-
  Sum1 : Sum  Inputs=|++
  cos30 : Constant  Value=cosd(30)
  g : Constant  Value=g
  m_sphere : Constant  Value=mS
  r_ABC : Constant  Value=rABC
  "d_phi " : Outport
  "phi " : Outport  Port=2
  wires:
  cos30/1 -> Product/2, Product1/1
  FB/1 -> Product/1
  FC/1 -> Product1/2
  Product/1 -> Sum/1
  Product1/1 -> Sum/2
  Sum/1 -> Product2/1
  r_ABC/1 -> Product2/2
  Product2/1 -> Sum1/1
  m_sphere/1 -> Product3/1
  g/1 -> Product3/2
  Product3/1 -> Product4/2
  Ys/1 -> Product4/1
  Product4/1 -> Sum1/2
  Sum1/1 -> Divide/1
  Constant/1 -> Divide/2
  Divide/1 -> Integrator/1
  Integrator/1 -> "d_phi "/1, Integrator1/1
  Integrator1/1 -> "phi "/1

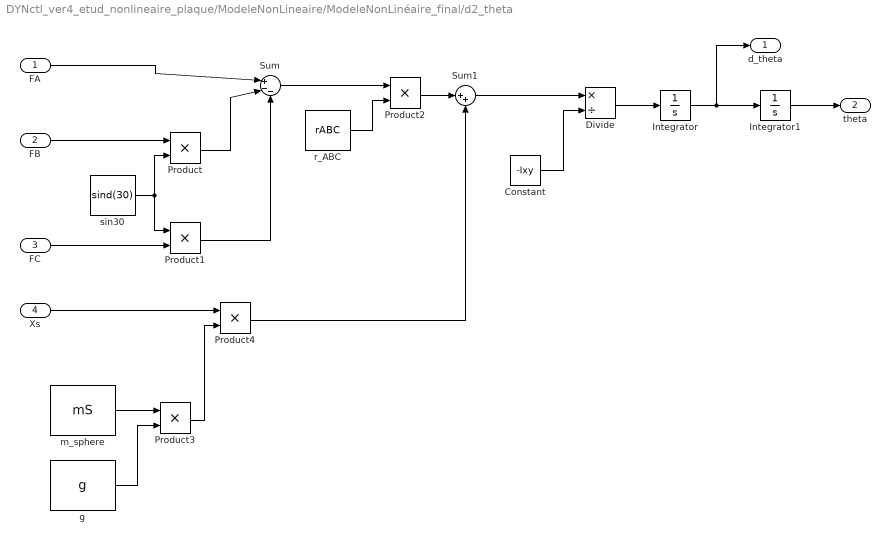
== system DYNctl_ver4_etud_nonlineaire_plaque/ModeleNonLineaire/ModeleNonLinéaire_final/d2_theta ==
  FA : Inport
  FB : Inport  Port=2
  FC : Inport  Port=3
  Xs : Inport  Port=4
  Constant : Constant  Value=-Ixy
  Divide : Product  Inputs=*/
  Integrator : Integrator
  Integrator1 : Integrator
  Product{,1..4} (5 alike) : Product
  Sum : Sum  Inputs=|+--
  Sum1 : Sum  Inputs=|++
  g : Constant  Value=g
  m_sphere : Constant  Value=mS
  r_ABC : Constant  Value=rABC
  sin30 : Constant  Value=sind(30)
  "d_theta " : Outport
  "theta " : Outport  Port=2
  wires:
  sin30/1 -> Product/2, Product1/1
  FB/1 -> Product/1
  FC/1 -> Product1/2
  FA/1 -> Sum/1
  Product/1 -> Sum/2
  Product1/1 -> Sum/3
  Sum/1 -> Product2/1
  r_ABC/1 -> Product2/2
  Product2/1 -> Sum1/1
  m_sphere/1 -> Product3/1
  g/1 -> Product3/2
  Product3/1 -> Product4/2
  Xs/1 -> Product4/1
  Product4/1 -> Sum1/2
  Sum1/1 -> Divide/1
  Constant/1 -> Divide/2
  Divide/1 -> Integrator/1
  Integrator/1 -> "d_theta "/1, Integrator1/1
  Integrator1/1 -> "theta "/1

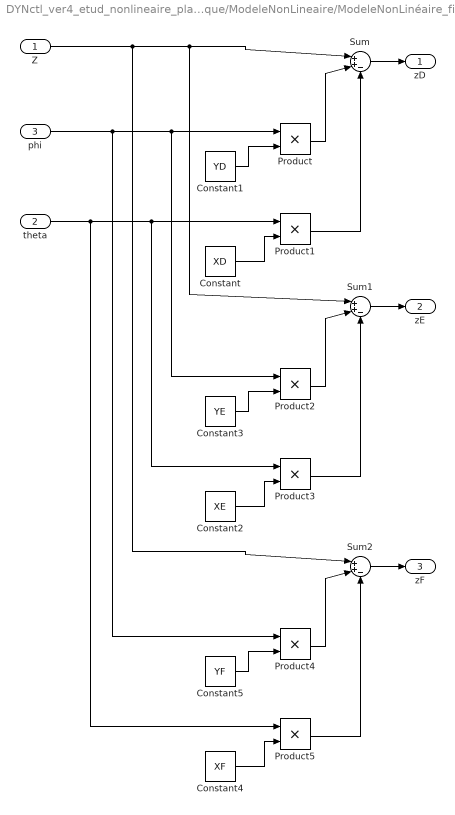
== system DYNctl_ver4_etud_nonlineaire_plaque/ModeleNonLineaire/ModeleNonLinéaire_final/dk ==
  Z : Inport
  theta : Inport  Port=2
  phi : Inport  Port=3
  Constant : Constant  Value=XD
  Constant1 : Constant  Value=YD
  Constant2 : Constant  Value=XE
  Constant3 : Constant  Value=YE
  Constant4 : Constant  Value=XF
  Constant5 : Constant  Value=YF
  Product{,1..5} (6 alike) : Product
  Sum : Sum  Inputs=|++-
  Sum1 : Sum  Inputs=|++-
  Sum2 : Sum  Inputs=|++-
  zD : Outport
  zE : Outport  Port=2
  zF : Outport  Port=3
  wires:
  Constant1/1 -> Product/2
  Product/1 -> Sum/2
  Constant/1 -> Product1/2
  Product1/1 -> Sum/3
  Sum/1 -> zD/1
  Constant3/1 -> Product2/2
  Product2/1 -> Sum1/2
  Constant2/1 -> Product3/2
  Product3/1 -> Sum1/3
  Sum1/1 -> zE/1
  phi/1 -> Product4/1, Product2/1, Product/1
  Constant5/1 -> Product4/2
  Product4/1 -> Sum2/2
  Z/1 -> Sum2/1, Sum1/1, Sum/1
  theta/1 -> Product5/1, Product3/1, Product1/1
  Constant4/1 -> Product5/2
  Product5/1 -> Sum2/3
  Sum2/1 -> zF/1
